simulink model "lab2_model_ssEmulation"  (R2024b)
settings: Solver=FixedStepAuto  StartTime=0.0  StopTime=sIn.simulation_time  FixedStep=sIn.step_size
values from neighbouring files (symbols this model uses):
  obsD = obs.tmp(sIn.integrationMethod)    [lab2_startup_ssEmulation.m]
undefined symbols (not defined in the file or in its folder): DiscIntNeverNeededParam, drv, feedback, gbox, mld, mot, obs, rads2rpm, rpm2rads, sens, sIn
libraries: simulink_extras x4, simulink x1
settings Model: Creator=bmm1  LastModifiedBy=pries
settings DataIOCC: ReturnWorkspaceOutputs=off
settings RTWCC: GPUComputeCapability=3.5

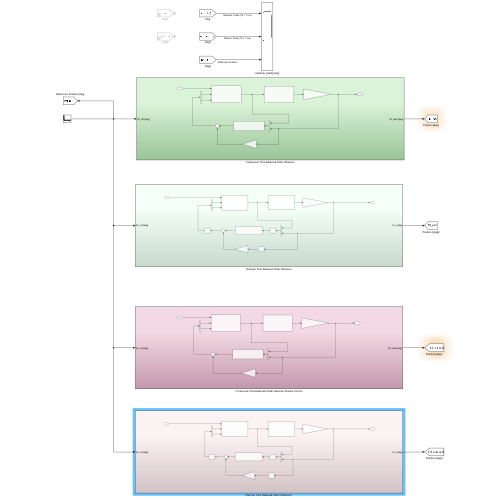
[thumbnail: Simulink's stored preview of the top-level diagram]
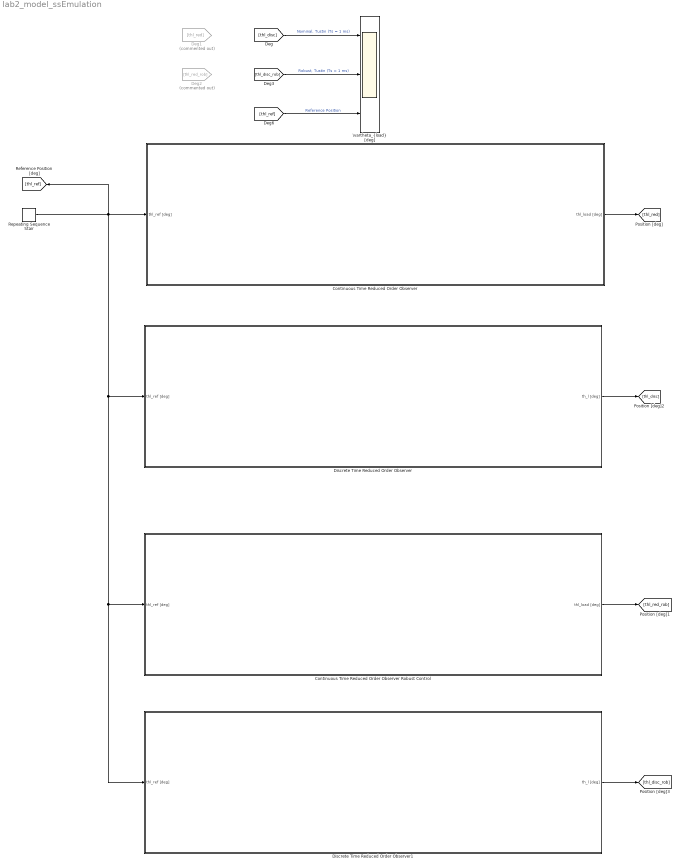
== system lab2_model_ssEmulation ==
  Continuous Time Reduced Order Observer : Subsystem
  Continuous Time Reduced Order Observer Robust Control : Subsystem
  Deg1 : From  Commented=on  GotoTag=thl_red
  Deg2 : From  Commented=on  GotoTag=thl_red_rob
  Discrete Time Reduced Order Observer : Subsystem
  Discrete Time Reduced Order Observer1 : Subsystem
  Repeating Sequence Stair : simulink/Sources/Repeating Sequence Stair  OutValues=sIn.position  tsamp=sIn.sample_time  OutMin=[]  OutMax=[]  OutDataTypeStr=double  OutputDataTypeScalingMode=double  OutDataType=fixdt(0,8)  ConRadixGroup=Best Precision: Vector-wise  OutScaling=2^-12
  "\\vartheta_{load} [deg]" : Scope  NumInputPorts=3
  wires:
  [thl_ref] -> "\\vartheta_{load} [deg]"/3  "Reference Position"
  Repeating Sequence Stair/1 -> Continuous Time Reduced Order Observer/1(thl_ref [deg]), Discrete Time Reduced Order Observer1/1(thl_ref [deg]), Continuous Time Reduced Order Observer Robust Control/1(thl_ref [deg]), Discrete Time Reduced Order Observer/1(thl_ref [deg]), [thl_ref]
  Continuous Time Reduced Order Observer/1(thl_load [deg]) -> [thl_red]
  Discrete Time Reduced Order Observer/1(th_l [deg]) -> [thl_disc]
  Continuous Time Reduced Order Observer Robust Control/1(thl_load [deg]) -> [thl_red_rob]
  Discrete Time Reduced Order Observer1/1(th_l [deg]) -> [thl_disc_rob]
  [thl_disc] -> "\\vartheta_{load} [deg]"/1  "Nominal, Tustin (Ts = 1 ms)"
  [thl_disc_rob] -> "\\vartheta_{load} [deg]"/2  "Robust, Tustin (Ts = 1 ms)"

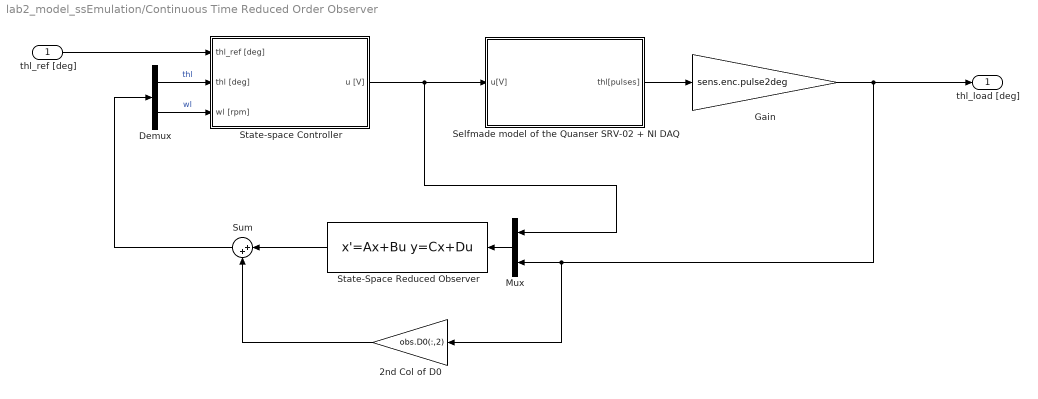
== system lab2_model_ssEmulation/Continuous Time Reduced Order Observer ==
  thl_ref [deg] : Inport
  2nd Col of D0 : Gain  Gain=obs.D0(:,2)
  Demux : Demux  Outputs=2
  Gain : Gain  Gain=sens.enc.pulse2deg
  Mux : Mux  Inputs=2
  Selfmade model of the Quanser SRV-02 + NI DAQ : Subsystem
  State-Space Reduced Observer : StateSpace  A=obs.A0  B=obs.B0  C=obs.C0  D=zeros(2,2)  InitialCondition=0
  State-space Controller : Subsystem
  Sum : Sum  Inputs=|++
  thl_load [deg] : Outport
  wires:
  Selfmade model of the Quanser SRV-02 + NI DAQ/1(thl[pulses]) -> Gain/1
  Gain/1 -> thl_load [deg]/1, 2nd Col of D0/1, Mux/2
  State-space Controller/1(u [V]) -> Mux/1, Selfmade model of the Quanser SRV-02 + NI DAQ/1(u[V])
  Demux/1 -> State-space Controller/2(thl [deg])  "thl"
  Mux/1 -> State-Space Reduced Observer/1
  Demux/2 -> State-space Controller/3(wl [rpm])  "wl"
  thl_ref [deg]/1 -> State-space Controller/1(thl_ref [deg])
  State-Space Reduced Observer/1 -> Sum/1
  Sum/1 -> Demux/1
  2nd Col of D0/1 -> Sum/2

== system lab2_model_ssEmulation/Continuous Time Reduced Order Observer Robust Control ==
  thl_ref [deg] : Inport
  2nd Col of D0 : Gain  Gain=obs.D0(:,2)
  Demux : Demux  Outputs=2
  Gain : Gain  Gain=sens.enc.pulse2deg
  Mux : Mux  Inputs=2
  Selfmade model of the Quanser SRV-02 + NI DAQ : Subsystem
  State-Space Reduced Observer : StateSpace  A=obs.A0  B=obs.B0  C=obs.C0  D=zeros(2,2)  InitialCondition=0
  State-space Controller : Subsystem
  Sum : Sum  Inputs=|++
  thl_load [deg] : Outport
  wires:
  Selfmade model of the Quanser SRV-02 + NI DAQ/1(thl[pulses]) -> Gain/1
  Gain/1 -> thl_load [deg]/1, 2nd Col of D0/1, Mux/2
  State-space Controller/1(u [V]) -> Mux/1, Selfmade model of the Quanser SRV-02 + NI DAQ/1(u[V])
  Demux/1 -> State-space Controller/2(thl [deg])  "thl"
  Mux/1 -> State-Space Reduced Observer/1
  Demux/2 -> State-space Controller/3(wl [rpm])  "wl"
  thl_ref [deg]/1 -> State-space Controller/1(thl_ref [deg])
  State-Space Reduced Observer/1 -> Sum/1
  2nd Col of D0/1 -> Sum/2
  Sum/1 -> Demux/1

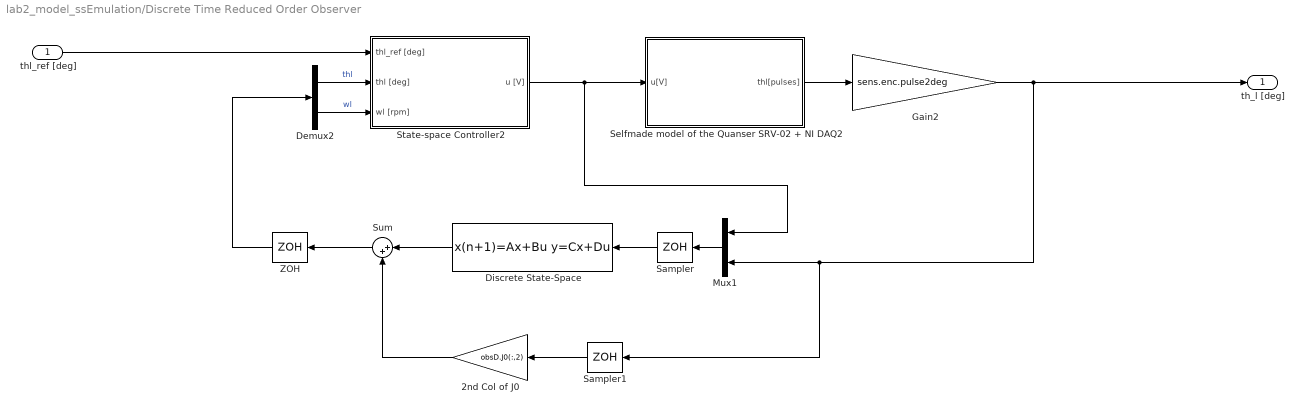
== system lab2_model_ssEmulation/Discrete Time Reduced Order Observer ==
  thl_ref [deg] : Inport
  2nd Col of J0 : Gain  Gain=obsD.J0(:,2)
  Demux2 : Demux  Outputs=2
  Discrete State-Space : DiscreteStateSpace  A=obsD.Phi0  B=obsD.Gamma0  C=obsD.H0  D=[obsD.J0(:,1), zeros(2,1)]  SampleTime=sIn.Ts
  Gain2 : Gain  Gain=sens.enc.pulse2deg
  Mux1 : Mux  Inputs=2
  Sampler : ZeroOrderHold  SampleTime=sIn.Ts
  Sampler1 : ZeroOrderHold  SampleTime=sIn.Ts
  Selfmade model of the Quanser SRV-02 + NI DAQ2 : Subsystem
  State-space Controller2 : Subsystem
  Sum : Sum  Inputs=|++
  ZOH : ZeroOrderHold  SampleTime=sIn.Ts
  th_l [deg] : Outport
  wires:
  Sampler/1 -> Discrete State-Space/1
  Selfmade model of the Quanser SRV-02 + NI DAQ2/1(thl[pulses]) -> Gain2/1
  Mux1/1 -> Sampler/1
  State-space Controller2/1(u [V]) -> Selfmade model of the Quanser SRV-02 + NI DAQ2/1(u[V]), Mux1/1
  Demux2/2 -> State-space Controller2/3(wl [rpm])  "wl"
  Gain2/1 -> th_l [deg]/1, Sampler1/1, Mux1/2
  Demux2/1 -> State-space Controller2/2(thl [deg])  "thl"
  ZOH/1 -> Demux2/1
  thl_ref [deg]/1 -> State-space Controller2/1(thl_ref [deg])
  Sampler1/1 -> 2nd Col of J0/1
  Sum/1 -> ZOH/1
  Discrete State-Space/1 -> Sum/1
  2nd Col of J0/1 -> Sum/2

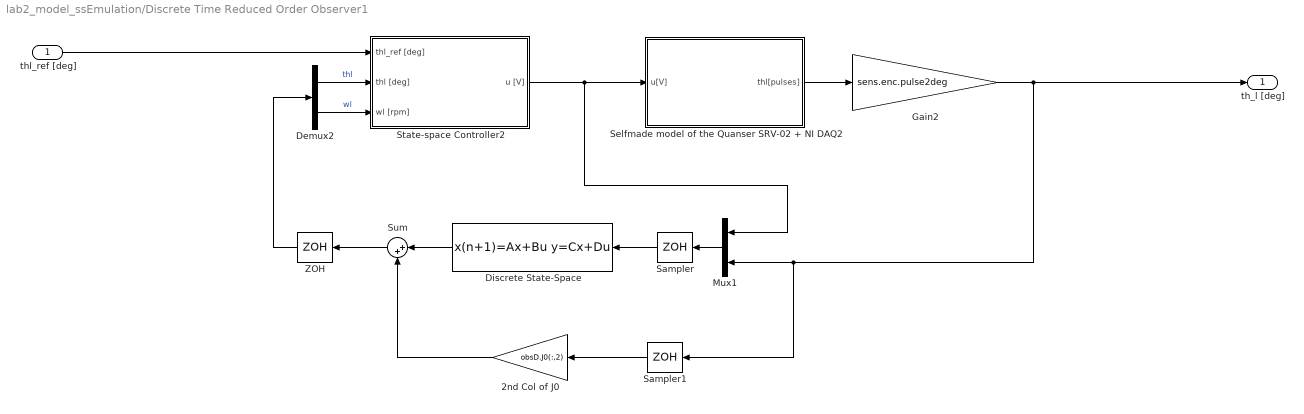
== system lab2_model_ssEmulation/Discrete Time Reduced Order Observer1 ==
  thl_ref [deg] : Inport
  2nd Col of J0 : Gain  Gain=obsD.J0(:,2)
  Demux2 : Demux  Outputs=2
  Discrete State-Space : DiscreteStateSpace  A=obsD.Phi0  B=obsD.Gamma0  C=obsD.H0  D=[obsD.J0(:,1), zeros(2,1)]  SampleTime=sIn.Ts
  Gain2 : Gain  Gain=sens.enc.pulse2deg
  Mux1 : Mux  Inputs=2
  Sampler : ZeroOrderHold  SampleTime=sIn.Ts
  Sampler1 : ZeroOrderHold  SampleTime=sIn.Ts
  Selfmade model of the Quanser SRV-02 + NI DAQ2 : Subsystem
  State-space Controller2 : Subsystem
  Sum : Sum  Inputs=|++
  ZOH : ZeroOrderHold  SampleTime=sIn.Ts
  th_l [deg] : Outport
  wires:
  thl_ref [deg]/1 -> State-space Controller2/1(thl_ref [deg])
  ZOH/1 -> Demux2/1
  Demux2/1 -> State-space Controller2/2(thl [deg])  "thl"
  Gain2/1 -> Sampler1/1, Mux1/2, th_l [deg]/1
  Demux2/2 -> State-space Controller2/3(wl [rpm])  "wl"
  State-space Controller2/1(u [V]) -> Mux1/1, Selfmade model of the Quanser SRV-02 + NI DAQ2/1(u[V])
  Mux1/1 -> Sampler/1
  Selfmade model of the Quanser SRV-02 + NI DAQ2/1(thl[pulses]) -> Gain2/1
  Sampler/1 -> Discrete State-Space/1
  Sampler1/1 -> 2nd Col of J0/1
  Sum/1 -> ZOH/1
  Discrete State-Space/1 -> Sum/1
  2nd Col of J0/1 -> Sum/2

== system lab2_model_ssEmulation/Continuous Time Reduced Order Observer/Selfmade model of the Quanser SRV-02 + NI DAQ ==
  u[V] : Inport
  DAC : Subsystem
  DC motor + gearbox : Subsystem
  Encoder : Subsystem
  Terminator : Terminator
  Terminator1 : Terminator
  Voltage driver : Subsystem
  thl[pulses] : Outport
  wires:
  DC motor + gearbox/1(thl[deg]) -> Encoder/1(thl[deg])  "Deg"
  u[V]/1 -> DAC/1(u[V])
  DC motor + gearbox/2(wl[rpm]) -> Terminator/1  "RPM"
  DAC/1(udrv[V]) -> Voltage driver/1(u[V])
  Voltage driver/1(udrv[v]) -> DC motor + gearbox/1(udrv[V])
  Encoder/1(thl[pulses]) -> thl[pulses]/1
  DC motor + gearbox/3(uRs [V]) -> Terminator1/1

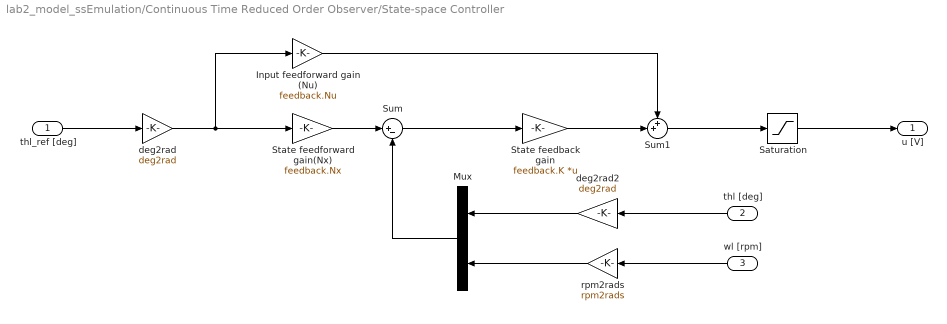
== system lab2_model_ssEmulation/Continuous Time Reduced Order Observer/State-space Controller ==
  thl_ref [deg] : Inport
  thl [deg] : Inport  Port=2
  wl [rpm] : Inport  Port=3
  Input feedforward gain (Nu) : Gain  Gain=feedback.Nu
  Mux : Mux  Inputs=2
  Saturation : Saturate  UpperLimit=10  LowerLimit=-10
  State feedback gain : Gain  Gain=feedback.K  Multiplication=Matrix(K*u)
  State feedforward gain(Nx) : Gain  Gain=feedback.Nx
  Sum : Sum  Inputs=|+-
  Sum1 : Sum  Inputs=++|
  deg2rad : Gain  Gain=deg2rad
  deg2rad2 : Gain  Gain=deg2rad
  rpm2rads : Gain  Gain=rpm2rads
  u [V] : Outport
  wires:
  thl_ref [deg]/1 -> deg2rad/1
  deg2rad/1 -> Input feedforward gain (Nu)/1, State feedforward gain(Nx)/1
  State feedforward gain(Nx)/1 -> Sum/1
  Sum/1 -> State feedback gain/1
  State feedback gain/1 -> Sum1/2
  Input feedforward gain (Nu)/1 -> Sum1/1
  Sum1/1 -> Saturation/1
  Saturation/1 -> u [V]/1
  thl [deg]/1 -> deg2rad2/1
  wl [rpm]/1 -> rpm2rads/1
  deg2rad2/1 -> Mux/1
  rpm2rads/1 -> Mux/2
  Mux/1 -> Sum/2

== system lab2_model_ssEmulation/Continuous Time Reduced Order Observer Robust Control/Selfmade model of the Quanser SRV-02 + NI DAQ ==
  u[V] : Inport
  DAC : Subsystem
  DC motor + gearbox : Subsystem
  Encoder : Subsystem
  Terminator : Terminator
  Terminator1 : Terminator
  Voltage driver : Subsystem
  thl[pulses] : Outport
  wires:
  DC motor + gearbox/1(thl[deg]) -> Encoder/1(thl[deg])  "Deg"
  u[V]/1 -> DAC/1(u[V])
  DC motor + gearbox/2(wl[rpm]) -> Terminator/1  "RPM"
  DAC/1(udrv[V]) -> Voltage driver/1(u[V])
  Voltage driver/1(udrv[v]) -> DC motor + gearbox/1(udrv[V])
  Encoder/1(thl[pulses]) -> thl[pulses]/1
  DC motor + gearbox/3(uRs [V]) -> Terminator1/1

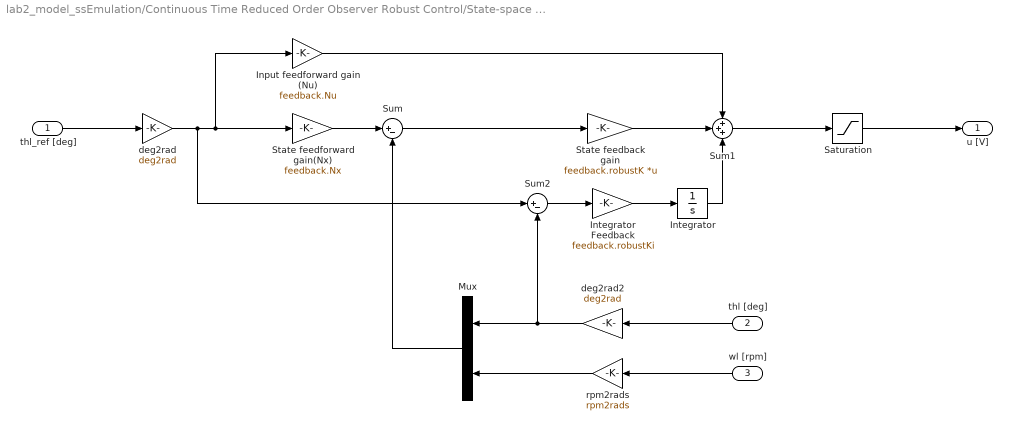
== system lab2_model_ssEmulation/Continuous Time Reduced Order Observer Robust Control/State-space Controller ==
  thl_ref [deg] : Inport
  thl [deg] : Inport  Port=2
  wl [rpm] : Inport  Port=3
  Input feedforward gain (Nu) : Gain  Gain=feedback.Nu
  Integrator : Integrator
  Integrator Feedback : Gain  Gain=feedback.robustKi
  Mux : Mux  Inputs=2
  Saturation : Saturate  UpperLimit=10  LowerLimit=-10
  State feedback gain : Gain  Gain=feedback.robustK  Multiplication=Matrix(K*u)
  State feedforward gain(Nx) : Gain  Gain=feedback.Nx
  Sum : Sum  Inputs=|+-
  Sum1 : Sum  Inputs=+++
  Sum2 : Sum  Inputs=|+-
  deg2rad : Gain  Gain=deg2rad
  deg2rad2 : Gain  Gain=deg2rad
  rpm2rads : Gain  Gain=rpm2rads
  u [V] : Outport
  wires:
  thl_ref [deg]/1 -> deg2rad/1
  deg2rad/1 -> Sum2/1, Input feedforward gain (Nu)/1, State feedforward gain(Nx)/1
  State feedforward gain(Nx)/1 -> Sum/1
  Sum/1 -> State feedback gain/1
  State feedback gain/1 -> Sum1/2
  Input feedforward gain (Nu)/1 -> Sum1/1
  Sum1/1 -> Saturation/1
  Saturation/1 -> u [V]/1
  thl [deg]/1 -> deg2rad2/1
  wl [rpm]/1 -> rpm2rads/1
  deg2rad2/1 -> Sum2/2, Mux/1
  rpm2rads/1 -> Mux/2
  Mux/1 -> Sum/2
  Integrator Feedback/1 -> Integrator/1
  Integrator/1 -> Sum1/3
  Sum2/1 -> Integrator Feedback/1

== system lab2_model_ssEmulation/Discrete Time Reduced Order Observer/Selfmade model of the Quanser SRV-02 + NI DAQ2 ==
  u[V] : Inport
  DAC : Subsystem
  DC motor + gearbox : Subsystem
  Encoder : Subsystem
  Terminator : Terminator
  Terminator1 : Terminator
  Voltage driver : Subsystem
  thl[pulses] : Outport
  wires:
  DC motor + gearbox/3(uRs [V]) -> Terminator1/1
  Encoder/1(thl[pulses]) -> thl[pulses]/1
  Voltage driver/1(udrv[v]) -> DC motor + gearbox/1(udrv[V])
  DAC/1(udrv[V]) -> Voltage driver/1(u[V])
  DC motor + gearbox/2(wl[rpm]) -> Terminator/1  "RPM"
  u[V]/1 -> DAC/1(u[V])
  DC motor + gearbox/1(thl[deg]) -> Encoder/1(thl[deg])  "Deg"

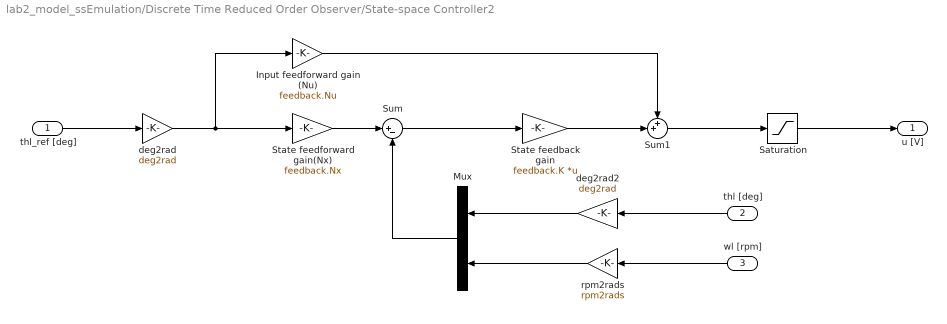
== system lab2_model_ssEmulation/Discrete Time Reduced Order Observer/State-space Controller2 ==
  thl_ref [deg] : Inport
  thl [deg] : Inport  Port=2
  wl [rpm] : Inport  Port=3
  Input feedforward gain (Nu) : Gain  Gain=feedback.Nu
  Mux : Mux  Inputs=2
  Saturation : Saturate  UpperLimit=10  LowerLimit=-10
  State feedback gain : Gain  Gain=feedback.K  Multiplication=Matrix(K*u)
  State feedforward gain(Nx) : Gain  Gain=feedback.Nx
  Sum : Sum  Inputs=|+-
  Sum1 : Sum  Inputs=++|
  deg2rad : Gain  Gain=deg2rad
  deg2rad2 : Gain  Gain=deg2rad
  rpm2rads : Gain  Gain=rpm2rads
  u [V] : Outport
  wires:
  Mux/1 -> Sum/2
  rpm2rads/1 -> Mux/2
  deg2rad2/1 -> Mux/1
  wl [rpm]/1 -> rpm2rads/1
  thl [deg]/1 -> deg2rad2/1
  Saturation/1 -> u [V]/1
  Sum1/1 -> Saturation/1
  Input feedforward gain (Nu)/1 -> Sum1/1
  State feedback gain/1 -> Sum1/2
  Sum/1 -> State feedback gain/1
  State feedforward gain(Nx)/1 -> Sum/1
  deg2rad/1 -> State feedforward gain(Nx)/1, Input feedforward gain (Nu)/1
  thl_ref [deg]/1 -> deg2rad/1

== system lab2_model_ssEmulation/Discrete Time Reduced Order Observer1/Selfmade model of the Quanser SRV-02 + NI DAQ2 ==
  u[V] : Inport
  DAC : Subsystem
  DC motor + gearbox : Subsystem
  Encoder : Subsystem
  Terminator : Terminator
  Terminator1 : Terminator
  Voltage driver : Subsystem
  thl[pulses] : Outport
  wires:
  DC motor + gearbox/1(thl[deg]) -> Encoder/1(thl[deg])  "Deg"
  u[V]/1 -> DAC/1(u[V])
  DC motor + gearbox/2(wl[rpm]) -> Terminator/1  "RPM"
  DAC/1(udrv[V]) -> Voltage driver/1(u[V])
  Voltage driver/1(udrv[v]) -> DC motor + gearbox/1(udrv[V])
  Encoder/1(thl[pulses]) -> thl[pulses]/1
  DC motor + gearbox/3(uRs [V]) -> Terminator1/1

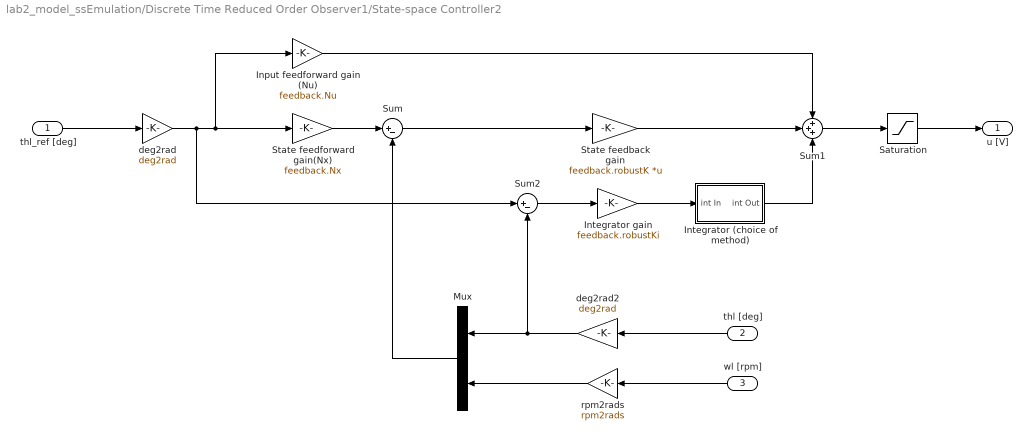
== system lab2_model_ssEmulation/Discrete Time Reduced Order Observer1/State-space Controller2 ==
  thl_ref [deg] : Inport
  thl [deg] : Inport  Port=2
  wl [rpm] : Inport  Port=3
  Input feedforward gain (Nu) : Gain  Gain=feedback.Nu
  Integrator (choice of method) : Subsystem
  Integrator gain : Gain  Gain=feedback.robustKi
  Mux : Mux  Inputs=2
  Saturation : Saturate  UpperLimit=10  LowerLimit=-10
  State feedback gain : Gain  Gain=feedback.robustK  Multiplication=Matrix(K*u)
  State feedforward gain(Nx) : Gain  Gain=feedback.Nx
  Sum : Sum  Inputs=|+-
  Sum1 : Sum  Inputs=+++
  Sum2 : Sum  Inputs=|+-
  deg2rad : Gain  Gain=deg2rad
  deg2rad2 : Gain  Gain=deg2rad
  rpm2rads : Gain  Gain=rpm2rads
  u [V] : Outport
  wires:
  thl_ref [deg]/1 -> deg2rad/1
  deg2rad/1 -> Sum2/1, Input feedforward gain (Nu)/1, State feedforward gain(Nx)/1
  State feedforward gain(Nx)/1 -> Sum/1
  Sum/1 -> State feedback gain/1
  State feedback gain/1 -> Sum1/2
  Input feedforward gain (Nu)/1 -> Sum1/1
  Sum1/1 -> Saturation/1
  Saturation/1 -> u [V]/1
  thl [deg]/1 -> deg2rad2/1
  wl [rpm]/1 -> rpm2rads/1
  deg2rad2/1 -> Sum2/2, Mux/1
  rpm2rads/1 -> Mux/2
  Mux/1 -> Sum/2
  Sum2/1 -> Integrator gain/1
  Integrator gain/1 -> Integrator (choice of method)/1(int In)
  Integrator (choice of method)/1(int Out) -> Sum1/3

== system lab2_model_ssEmulation/Continuous Time Reduced Order Observer/Selfmade model of the Quanser SRV-02 + NI DAQ/DAC ==
  u[V] : Inport
  Quantizer : Quantizer  QuantizationInterval=daq.dac.q
  Saturation : Saturate  UpperLimit=10  LowerLimit=-10
  Zero-Order Hold : ZeroOrderHold  SampleTime=1e-3
  udrv[V] : Outport
  wires:
  Zero-Order Hold/1 -> Quantizer/1
  u[V]/1 -> Zero-Order Hold/1
  Quantizer/1 -> Saturation/1
  Saturation/1 -> udrv[V]/1

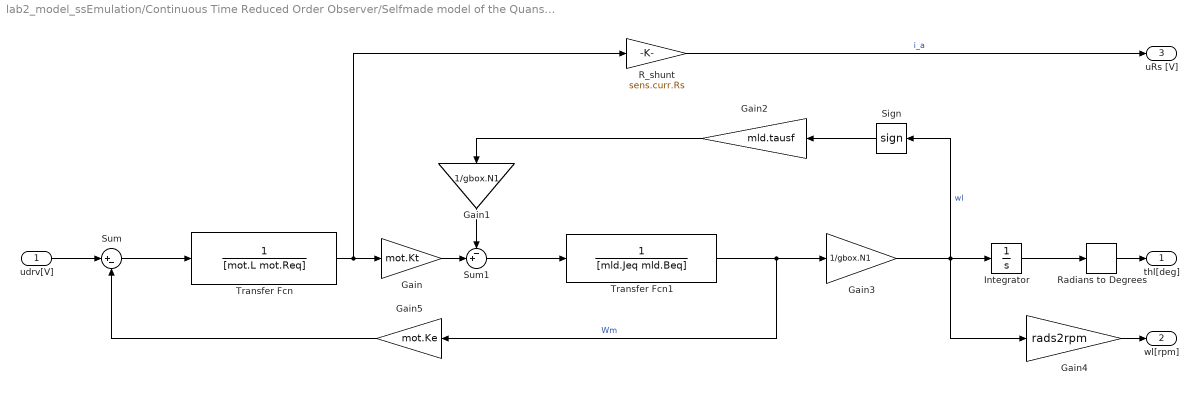
== system lab2_model_ssEmulation/Continuous Time Reduced Order Observer/Selfmade model of the Quanser SRV-02 + NI DAQ/DC motor + gearbox ==
  udrv[V] : Inport
  Gain : Gain  Gain=mot.Kt
  Gain1 : Gain  Gain=1/gbox.N1
  Gain2 : Gain  Gain=mld.tausf
  Gain3 : Gain  Gain=1/gbox.N1
  Gain4 : Gain  Gain=rads2rpm
  Gain5 : Gain  Gain=mot.Ke
  Integrator : Integrator
  R_shunt : Gain  Gain=sens.curr.Rs
  Radians to Degrees : simulink_extras/Transformations/Radians to Degrees
  Sign : Signum  ZeroCross=off
  Sum : Sum  Inputs=|+-
  Sum1 : Sum  Inputs=-+|
  Transfer Fcn : TransferFcn  Denominator=[mot.L mot.Req]
  Transfer Fcn1 : TransferFcn  Denominator=[mld.Jeq mld.Beq]
  thl[deg] : Outport
  wl[rpm] : Outport  Port=2
  uRs [V] : Outport  Port=3
  wires:
  udrv[V]/1 -> Sum/1
  Sum/1 -> Transfer Fcn/1
  Transfer Fcn/1 -> R_shunt/1, Gain/1
  Gain1/1 -> Sum1/1
  Gain2/1 -> Gain1/1
  Sign/1 -> Gain2/1
  Transfer Fcn1/1 -> Gain5/1, Gain3/1  "Wm"
  Gain3/1 -> Gain4/1, Sign/1, Integrator/1  "wl"
  Integrator/1 -> Radians to Degrees/1
  Radians to Degrees/1 -> thl[deg]/1
  Gain4/1 -> wl[rpm]/1
  Sum1/1 -> Transfer Fcn1/1
  Gain/1 -> Sum1/2
  Gain5/1 -> Sum/2
  R_shunt/1 -> uRs [V]/1  "i_a"

== system lab2_model_ssEmulation/Continuous Time Reduced Order Observer/Selfmade model of the Quanser SRV-02 + NI DAQ/Encoder ==
  thl[deg] : Inport
  Gain : Gain  Gain=1/sens.enc.pulse2deg
  Quantizer : Quantizer  QuantizationInterval=sens.enc.pulse2deg
  Zero-Order Hold : ZeroOrderHold  SampleTime=1e-3
  thl[pulses] : Outport
  wires:
  thl[deg]/1 -> Zero-Order Hold/1
  Gain/1 -> thl[pulses]/1
  Quantizer/1 -> Gain/1
  Zero-Order Hold/1 -> Quantizer/1

== system lab2_model_ssEmulation/Continuous Time Reduced Order Observer/Selfmade model of the Quanser SRV-02 + NI DAQ/Voltage driver ==
  u[V] : Inport
  Saturation : Saturate  UpperLimit=12  LowerLimit=-12
  Transfer Fcn : TransferFcn  Numerator=[drv.dcgain]  Denominator=[drv.Tc 1]
  udrv[v] : Outport
  wires:
  u[V]/1 -> Transfer Fcn/1
  Transfer Fcn/1 -> Saturation/1
  Saturation/1 -> udrv[v]/1

== system lab2_model_ssEmulation/Continuous Time Reduced Order Observer Robust Control/Selfmade model of the Quanser SRV-02 + NI DAQ/DAC ==
  u[V] : Inport
  Quantizer : Quantizer  QuantizationInterval=daq.dac.q
  Saturation : Saturate  UpperLimit=10  LowerLimit=-10
  Zero-Order Hold : ZeroOrderHold  SampleTime=1e-3
  udrv[V] : Outport
  wires:
  Zero-Order Hold/1 -> Quantizer/1
  u[V]/1 -> Zero-Order Hold/1
  Quantizer/1 -> Saturation/1
  Saturation/1 -> udrv[V]/1

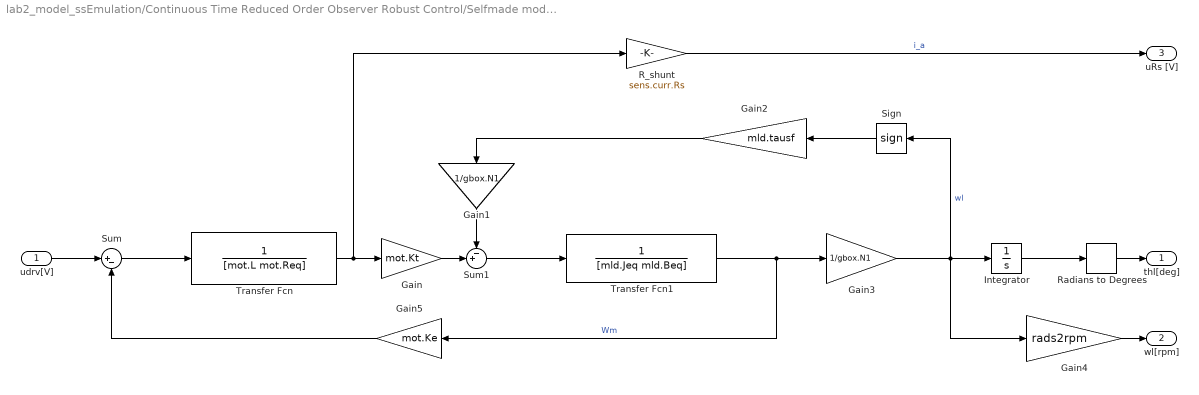
== system lab2_model_ssEmulation/Continuous Time Reduced Order Observer Robust Control/Selfmade model of the Quanser SRV-02 + NI DAQ/DC motor + gearbox ==
  udrv[V] : Inport
  Gain : Gain  Gain=mot.Kt
  Gain1 : Gain  Gain=1/gbox.N1
  Gain2 : Gain  Gain=mld.tausf
  Gain3 : Gain  Gain=1/gbox.N1
  Gain4 : Gain  Gain=rads2rpm
  Gain5 : Gain  Gain=mot.Ke
  Integrator : Integrator
  R_shunt : Gain  Gain=sens.curr.Rs
  Radians to Degrees : simulink_extras/Transformations/Radians to Degrees
  Sign : Signum  ZeroCross=off
  Sum : Sum  Inputs=|+-
  Sum1 : Sum  Inputs=-+|
  Transfer Fcn : TransferFcn  Denominator=[mot.L mot.Req]
  Transfer Fcn1 : TransferFcn  Denominator=[mld.Jeq mld.Beq]
  thl[deg] : Outport
  wl[rpm] : Outport  Port=2
  uRs [V] : Outport  Port=3
  wires:
  udrv[V]/1 -> Sum/1
  Sum/1 -> Transfer Fcn/1
  Transfer Fcn/1 -> R_shunt/1, Gain/1
  Gain1/1 -> Sum1/1
  Gain2/1 -> Gain1/1
  Sign/1 -> Gain2/1
  Transfer Fcn1/1 -> Gain5/1, Gain3/1  "Wm"
  Gain3/1 -> Gain4/1, Sign/1, Integrator/1  "wl"
  Integrator/1 -> Radians to Degrees/1
  Radians to Degrees/1 -> thl[deg]/1
  Gain4/1 -> wl[rpm]/1
  Sum1/1 -> Transfer Fcn1/1
  Gain/1 -> Sum1/2
  Gain5/1 -> Sum/2
  R_shunt/1 -> uRs [V]/1  "i_a"

== system lab2_model_ssEmulation/Continuous Time Reduced Order Observer Robust Control/Selfmade model of the Quanser SRV-02 + NI DAQ/Encoder ==
  thl[deg] : Inport
  Gain : Gain  Gain=1/sens.enc.pulse2deg
  Quantizer : Quantizer  QuantizationInterval=sens.enc.pulse2deg
  Zero-Order Hold : ZeroOrderHold  SampleTime=1e-3
  thl[pulses] : Outport
  wires:
  thl[deg]/1 -> Zero-Order Hold/1
  Gain/1 -> thl[pulses]/1
  Quantizer/1 -> Gain/1
  Zero-Order Hold/1 -> Quantizer/1

== system lab2_model_ssEmulation/Continuous Time Reduced Order Observer Robust Control/Selfmade model of the Quanser SRV-02 + NI DAQ/Voltage driver ==
  u[V] : Inport
  Saturation : Saturate  UpperLimit=12  LowerLimit=-12
  Transfer Fcn : TransferFcn  Numerator=[drv.dcgain]  Denominator=[drv.Tc 1]
  udrv[v] : Outport
  wires:
  u[V]/1 -> Transfer Fcn/1
  Transfer Fcn/1 -> Saturation/1
  Saturation/1 -> udrv[v]/1

== system lab2_model_ssEmulation/Discrete Time Reduced Order Observer/Selfmade model of the Quanser SRV-02 + NI DAQ2/DAC ==
  u[V] : Inport
  Quantizer : Quantizer  QuantizationInterval=daq.dac.q
  Saturation : Saturate  UpperLimit=10  LowerLimit=-10
  Zero-Order Hold : ZeroOrderHold  SampleTime=1e-3
  udrv[V] : Outport
  wires:
  Saturation/1 -> udrv[V]/1
  Quantizer/1 -> Saturation/1
  u[V]/1 -> Zero-Order Hold/1
  Zero-Order Hold/1 -> Quantizer/1

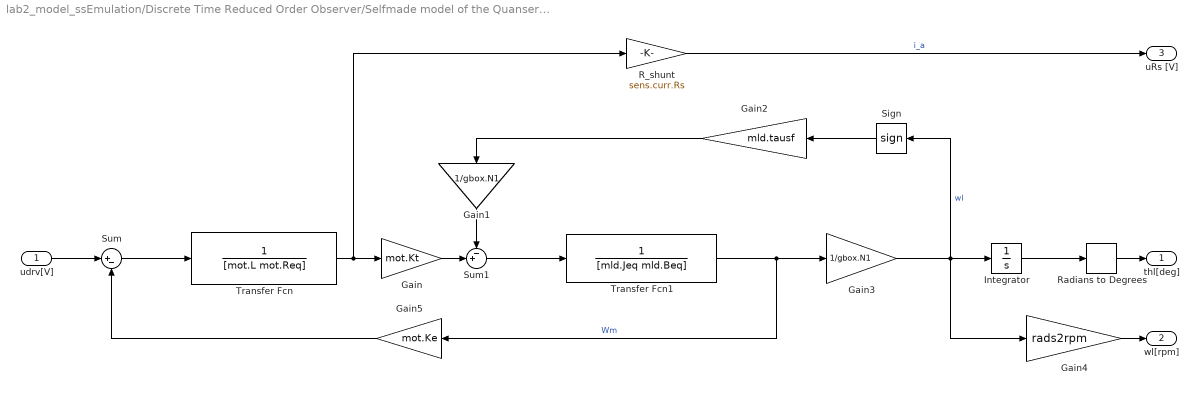
== system lab2_model_ssEmulation/Discrete Time Reduced Order Observer/Selfmade model of the Quanser SRV-02 + NI DAQ2/DC motor + gearbox ==
  udrv[V] : Inport
  Gain : Gain  Gain=mot.Kt
  Gain1 : Gain  Gain=1/gbox.N1
  Gain2 : Gain  Gain=mld.tausf
  Gain3 : Gain  Gain=1/gbox.N1
  Gain4 : Gain  Gain=rads2rpm
  Gain5 : Gain  Gain=mot.Ke
  Integrator : Integrator
  R_shunt : Gain  Gain=sens.curr.Rs
  Radians to Degrees : simulink_extras/Transformations/Radians to Degrees
  Sign : Signum  ZeroCross=off
  Sum : Sum  Inputs=|+-
  Sum1 : Sum  Inputs=-+|
  Transfer Fcn : TransferFcn  Denominator=[mot.L mot.Req]
  Transfer Fcn1 : TransferFcn  Denominator=[mld.Jeq mld.Beq]
  thl[deg] : Outport
  wl[rpm] : Outport  Port=2
  uRs [V] : Outport  Port=3
  wires:
  R_shunt/1 -> uRs [V]/1  "i_a"
  Gain5/1 -> Sum/2
  Gain/1 -> Sum1/2
  Sum1/1 -> Transfer Fcn1/1
  Gain4/1 -> wl[rpm]/1
  Radians to Degrees/1 -> thl[deg]/1
  Integrator/1 -> Radians to Degrees/1
  Gain3/1 -> Integrator/1, Sign/1, Gain4/1  "wl"
  Transfer Fcn1/1 -> Gain3/1, Gain5/1  "Wm"
  Sign/1 -> Gain2/1
  Gain2/1 -> Gain1/1
  Gain1/1 -> Sum1/1
  Transfer Fcn/1 -> Gain/1, R_shunt/1
  Sum/1 -> Transfer Fcn/1
  udrv[V]/1 -> Sum/1

== system lab2_model_ssEmulation/Discrete Time Reduced Order Observer/Selfmade model of the Quanser SRV-02 + NI DAQ2/Encoder ==
  thl[deg] : Inport
  Gain : Gain  Gain=1/sens.enc.pulse2deg
  Quantizer : Quantizer  QuantizationInterval=sens.enc.pulse2deg
  Zero-Order Hold : ZeroOrderHold  SampleTime=1e-3
  thl[pulses] : Outport
  wires:
  Zero-Order Hold/1 -> Quantizer/1
  Quantizer/1 -> Gain/1
  Gain/1 -> thl[pulses]/1
  thl[deg]/1 -> Zero-Order Hold/1

== system lab2_model_ssEmulation/Discrete Time Reduced Order Observer/Selfmade model of the Quanser SRV-02 + NI DAQ2/Voltage driver ==
  u[V] : Inport
  Saturation : Saturate  UpperLimit=12  LowerLimit=-12
  Transfer Fcn : TransferFcn  Numerator=[drv.dcgain]  Denominator=[drv.Tc 1]
  udrv[v] : Outport
  wires:
  Saturation/1 -> udrv[v]/1
  Transfer Fcn/1 -> Saturation/1
  u[V]/1 -> Transfer Fcn/1

== system lab2_model_ssEmulation/Discrete Time Reduced Order Observer1/Selfmade model of the Quanser SRV-02 + NI DAQ2/DAC ==
  u[V] : Inport
  Quantizer : Quantizer  QuantizationInterval=daq.dac.q
  Saturation : Saturate  UpperLimit=10  LowerLimit=-10
  Zero-Order Hold : ZeroOrderHold  SampleTime=1e-3
  udrv[V] : Outport
  wires:
  Zero-Order Hold/1 -> Quantizer/1
  u[V]/1 -> Zero-Order Hold/1
  Quantizer/1 -> Saturation/1
  Saturation/1 -> udrv[V]/1

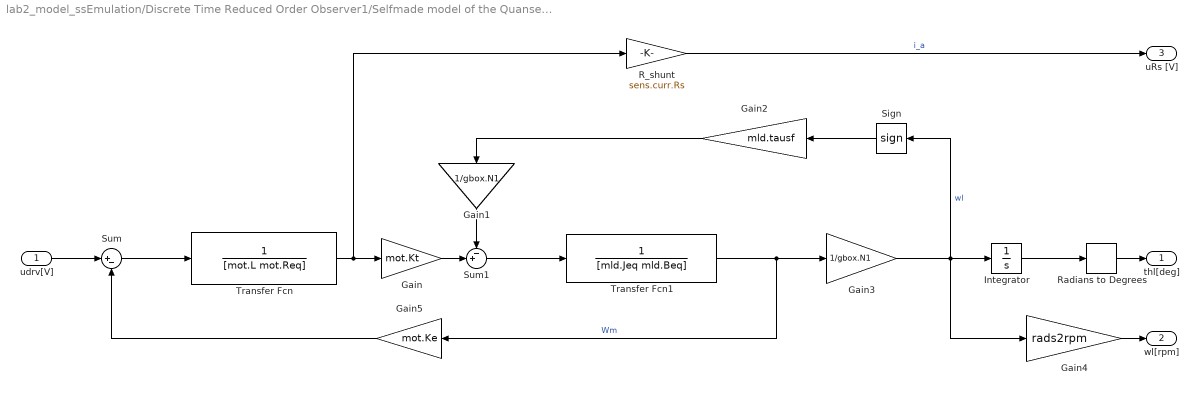
== system lab2_model_ssEmulation/Discrete Time Reduced Order Observer1/Selfmade model of the Quanser SRV-02 + NI DAQ2/DC motor + gearbox ==
  udrv[V] : Inport
  Gain : Gain  Gain=mot.Kt
  Gain1 : Gain  Gain=1/gbox.N1
  Gain2 : Gain  Gain=mld.tausf
  Gain3 : Gain  Gain=1/gbox.N1
  Gain4 : Gain  Gain=rads2rpm
  Gain5 : Gain  Gain=mot.Ke
  Integrator : Integrator
  R_shunt : Gain  Gain=sens.curr.Rs
  Radians to Degrees : simulink_extras/Transformations/Radians to Degrees
  Sign : Signum  ZeroCross=off
  Sum : Sum  Inputs=|+-
  Sum1 : Sum  Inputs=-+|
  Transfer Fcn : TransferFcn  Denominator=[mot.L mot.Req]
  Transfer Fcn1 : TransferFcn  Denominator=[mld.Jeq mld.Beq]
  thl[deg] : Outport
  wl[rpm] : Outport  Port=2
  uRs [V] : Outport  Port=3
  wires:
  udrv[V]/1 -> Sum/1
  Sum/1 -> Transfer Fcn/1
  Transfer Fcn/1 -> R_shunt/1, Gain/1
  Gain1/1 -> Sum1/1
  Gain2/1 -> Gain1/1
  Sign/1 -> Gain2/1
  Transfer Fcn1/1 -> Gain5/1, Gain3/1  "Wm"
  Gain3/1 -> Gain4/1, Sign/1, Integrator/1  "wl"
  Integrator/1 -> Radians to Degrees/1
  Radians to Degrees/1 -> thl[deg]/1
  Gain4/1 -> wl[rpm]/1
  Sum1/1 -> Transfer Fcn1/1
  Gain/1 -> Sum1/2
  Gain5/1 -> Sum/2
  R_shunt/1 -> uRs [V]/1  "i_a"

== system lab2_model_ssEmulation/Discrete Time Reduced Order Observer1/Selfmade model of the Quanser SRV-02 + NI DAQ2/Encoder ==
  thl[deg] : Inport
  Gain : Gain  Gain=1/sens.enc.pulse2deg
  Quantizer : Quantizer  QuantizationInterval=sens.enc.pulse2deg
  Zero-Order Hold : ZeroOrderHold  SampleTime=1e-3
  thl[pulses] : Outport
  wires:
  thl[deg]/1 -> Zero-Order Hold/1
  Gain/1 -> thl[pulses]/1
  Quantizer/1 -> Gain/1
  Zero-Order Hold/1 -> Quantizer/1

== system lab2_model_ssEmulation/Discrete Time Reduced Order Observer1/Selfmade model of the Quanser SRV-02 + NI DAQ2/Voltage driver ==
  u[V] : Inport
  Saturation : Saturate  UpperLimit=12  LowerLimit=-12
  Transfer Fcn : TransferFcn  Numerator=[drv.dcgain]  Denominator=[drv.Tc 1]
  udrv[v] : Outport
  wires:
  u[V]/1 -> Transfer Fcn/1
  Transfer Fcn/1 -> Saturation/1
  Saturation/1 -> udrv[v]/1

== system lab2_model_ssEmulation/Discrete Time Reduced Order Observer1/State-space Controller2/Integrator (choice of method) ==
  int In : Inport
  Backward Euler : DiscreteIntegrator  IntegratorMethod=Integration: Backward Euler  SampleTime=sIn.Ts  ICPrevOutput=DiscIntNeverNeededParam  ICPrevScaledInput=DiscIntNeverNeededParam
  Constant : Constant  Value=sIn.integrationMethod
  Forward Euler : DiscreteIntegrator  SampleTime=sIn.Ts  ICPrevOutput=DiscIntNeverNeededParam  ICPrevScaledInput=DiscIntNeverNeededParam
  Multiport Switch : MultiPortSwitch  SaturateOnIntegerOverflow=off  InputSameDT=off
  Tustin : DiscreteIntegrator  IntegratorMethod=Integration: Trapezoidal  SampleTime=sIn.Ts  ICPrevOutput=DiscIntNeverNeededParam  ICPrevScaledInput=DiscIntNeverNeededParam
  int Out : Outport
  wires:
  Forward Euler/1 -> Multiport Switch/2
  Backward Euler/1 -> Multiport Switch/3
  Tustin/1 -> Multiport Switch/4
  int In/1 -> Tustin/1, Forward Euler/1, Backward Euler/1
  Constant/1 -> Multiport Switch/1
  Multiport Switch/1 -> int Out/1
